simulink model "AircraftModel_LonMot_SAS"  (R2023b)
settings: Solver=VariableStepAuto  StartTime=0.0  StopTime=150  FixedStep=CNT_StepSize  RelTol=1e-3
undefined symbols (not defined in the file or in its folder): Actuators, CNT_g, CNT_m, ControlLaws, Propulsion, TestSequence, TrimPoint
libraries: simulink x6, vrlib x2
settings Model: Creator=NicolasS  LastModifiedBy=rouve
settings SolverCC: AlgebraicLoopSolver=TrustRegion
settings DataIOCC: ExternalInput=getinputstruct(TrimState_1_Op)  InitialState=getstatestruct(TrimState_1_Op)
settings DebuggingCC: UnconnectedInputMsg=warning  UnconnectedOutputMsg=warning  UnconnectedLineMsg=warning
settings ModelReferenceCC: EnableRefExpFcnMdlSchedulingChecks=on
settings RTWCC: DLArmComputeVersion=19.05

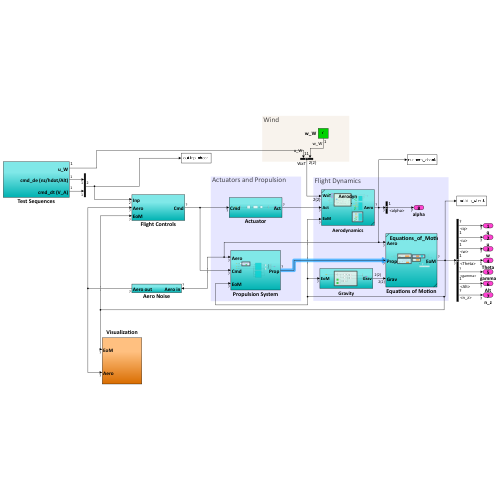
[thumbnail: Simulink's stored preview of the top-level diagram]
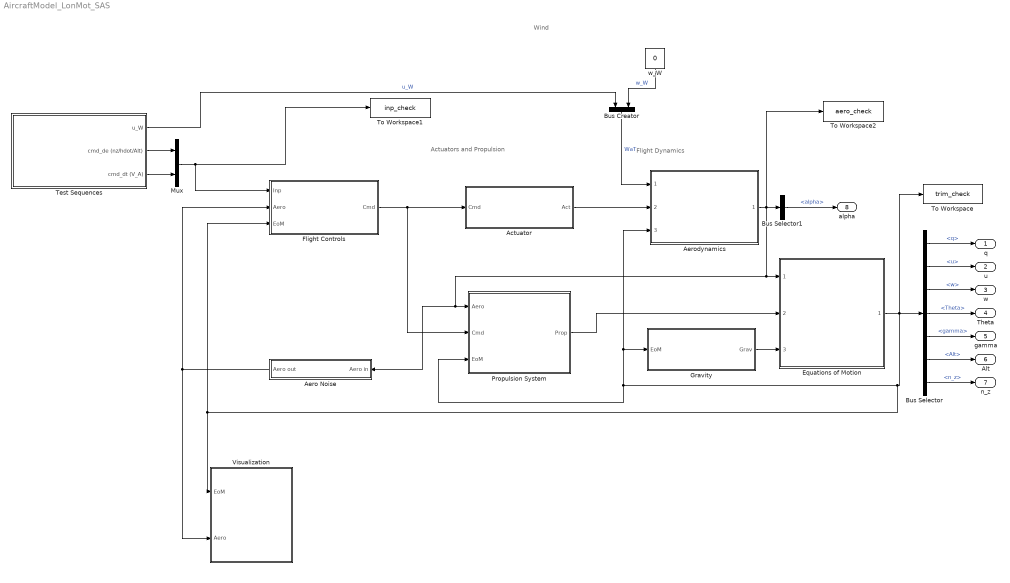
== system AircraftModel_LonMot_SAS ==
  note: Wind
  note: Actuators and Propulsion
  note: Flight Dynamics
  Actuator : Subsystem
  Aero Noise : Subsystem
  Aerodynamics : Subsystem  ReferencedSubsystem=Aerodyn
  Bus Creator : BusCreator  Inputs=2  OutDataTypeStr=Bus: WaT
  Bus Selector : BusSelector  OutputSignals=q,vv_f.u,vv_f.w,Theta,gamma,Alt,nn_f.n_z
  Bus Selector1 : BusSelector  OutputSignals=AirData.alpha
  Equations of Motion : Subsystem  ReferencedSubsystem=Equations_of_Motion
  Flight Controls : Subsystem
  Gravity : Subsystem
  Mux : Mux  Inputs=2
  Propulsion System : Subsystem
  Test Sequences : Subsystem  InitFcn=|  StopFcn=clear TestSequence
      | if not(exist('TestSequence','var'))
      |        TestSequence = 0;
      | end
  To Workspace : ToWorkspace  VariableName=trim_check  SaveFormat=Timeseries  SampleTime=-1
      settings: Decimation=2
  To Workspace1 : ToWorkspace  VariableName=inp_check  SaveFormat=Timeseries  SampleTime=-1
  To Workspace2 : ToWorkspace  VariableName=aero_check  SaveFormat=Timeseries  SampleTime=-1
  Visualization : Subsystem
  w_W : Constant  Value=0  SampleTime=-1
  q : Outport
  u : Outport  Port=2
  w : Outport  Port=3
  Theta : Outport  Port=4
  gamma : Outport  Port=5
  Alt : Outport  Port=6
  n_z : Outport  Port=7
  alpha : Outport  Port=8
  wires:
  Test Sequences/1(u_W) -> Bus Creator/1  "u_W"
  Bus Creator/1 -> Aerodynamics/1  "WaT"
  Actuator/1(Act) -> Aerodynamics/2
  Aerodynamics/1 -> To Workspace2/1, Bus Selector1/1, Propulsion System/1(Aero), Aero Noise/1(Aero in), Equations of Motion/1
  w_W/1 -> Bus Creator/2  "w_W"
  Propulsion System/1(Prop) -> Equations of Motion/2
  Bus Selector/6 -> Alt/1  "<Alt>"
  Bus Selector/1 -> q/1  "<q>"
  Bus Selector/2 -> u/1  "<u>"
  Bus Selector/3 -> w/1  "<w>"
  Bus Selector/4 -> Theta/1  "<Theta>"
  Bus Selector/7 -> n_z/1  "<n_z>"
  Bus Selector1/1 -> alpha/1  "<alpha>"
  Gravity/1(Grav) -> Equations of Motion/3
  Bus Selector/5 -> gamma/1  "<gamma>"
  Aero Noise/1(Aero out) -> Visualization/2(Aero), Flight Controls/2(Aero)
  Test Sequences/2(cmd_de (nz/hdot/Alt)) -> Mux/1
  Test Sequences/3(cmd_dt (V_A)) -> Mux/2
  Mux/1 -> Flight Controls/1(Inp), To Workspace1/1
  Flight Controls/1(Cmd) -> Propulsion System/2(Cmd), Actuator/1(Cmd)
  Equations of Motion/1 -> To Workspace/1, Visualization/1(EoM), Flight Controls/3(EoM), Propulsion System/3(EoM), Aerodynamics/3, Gravity/1(EoM), Bus Selector/1

== system AircraftModel_LonMot_SAS/Actuator ==
  Cmd : Inport  OutDataTypeStr=Bus: Cmd
  Bus Creator : BusCreator  Inputs=1  OutDataTypeStr=Bus: Act
  Bus Selector : BusSelector  OutputSignals=cmd_de
  Saturation : Saturate  UpperLimit=Actuators.Limits.u_max_He(2)  LowerLimit=Actuators.Limits.u_max_He(1)
  State-Space : StateSpace  A=Actuators.Act_e.A  B=Actuators.Act_e.B  C=Actuators.Act_e.C  D=Actuators.Act_e.D  InitialCondition=TrimPoint.States.debar  ParameterTunability=Unconstrained  ContinuousStateAttributes='de'
  Transport Delay : TransportDelay  DelayTime=0.04  InitialOutput=TrimPoint.States.debar  TransDelayFeedthrough=on
  Act : Outport  OutDataTypeStr=Bus: Act
  wires:
  Bus Creator/1 -> Act/1  "Act"
  Cmd/1 -> Bus Selector/1
  State-Space/1 -> Saturation/1  "de"
  Bus Selector/1 -> Transport Delay/1  "<cmd_de>"
  Saturation/1 -> Bus Creator/1  "de"
  Transport Delay/1 -> State-Space/1

== system AircraftModel_LonMot_SAS/Aero Noise ==
  Aero in : Inport  OutDataTypeStr=Bus: Aero
  Band-Limited White Noise8 : simulink/Sources/Band-Limited White Noise  Cov=1E-7  Ts=0.01  seed=3324
  Band-Limited White Noise9 : simulink/Sources/Band-Limited White Noise  Cov=1E-3  Ts=0.05  seed=8153
  Bus Creator2 : BusCreator  Inputs=4  OutDataTypeStr=Bus: Aero
  Bus Creator3 : BusCreator  Inputs=5  OutDataTypeStr=Bus: AirData
  Bus Selector : BusSelector  OutputSignals=AirData.u_Af,AirData.w_Af,AirData.V_A,AirData.p_dyn,AirData.alpha,X_Af,Z_Af,M_Af
  Sum1 : Sum  Inputs=++|
  Sum3 : Sum  Inputs=++|
  Aero out : Outport  OutDataTypeStr=Bus: Aero
  wires:
  Aero in/1 -> Bus Selector/1
  Bus Creator3/1 -> Bus Creator2/1  "AirData"
  Bus Selector/6 -> Bus Creator2/2  "<X_Af>"
  Bus Selector/7 -> Bus Creator2/3  "<Z_Af>"
  Bus Selector/8 -> Bus Creator2/4  "<M_Af>"
  Bus Creator2/1 -> Aero out/1  "Aero"
  Bus Selector/1 -> Bus Creator3/1  "<u_Af>"
  Bus Selector/2 -> Bus Creator3/2  "<w_Af>"
  Bus Selector/3 -> Sum3/2  "<V_A>"
  Bus Selector/5 -> Sum1/2  "<alpha>"
  Band-Limited White Noise8/1 -> Sum1/1
  Sum1/1 -> Bus Creator3/5  "alpha"
  Bus Selector/4 -> Bus Creator3/4  "<p_dyn>"
  Band-Limited White Noise9/1 -> Sum3/1
  Sum3/1 -> Bus Creator3/3  "V_A"

== system AircraftModel_LonMot_SAS/Flight Controls ==
  Inp : Inport
  Aero : Inport  Port=2  OutDataTypeStr=Bus: Aero
  EoM : Inport  Port=3  OutDataTypeStr=Bus: EoM
  Bus Creator2 : BusCreator  Inputs=2  OutDataTypeStr=Bus: Cmd
  Longitudinal Control Laws : Subsystem
  Cmd : Outport
  wires:
  EoM/1 -> Longitudinal Control Laws/2(EoM)
  Bus Creator2/1 -> Cmd/1  "Cmd"
  Longitudinal Control Laws/2(cmd_dt) -> Bus Creator2/2  "cmd_dt"
  Longitudinal Control Laws/1(cmd_de) -> Bus Creator2/1  "cmd_de"
  Inp/1 -> Longitudinal Control Laws/3(Inp)
  Aero/1 -> Longitudinal Control Laws/1(Aero)

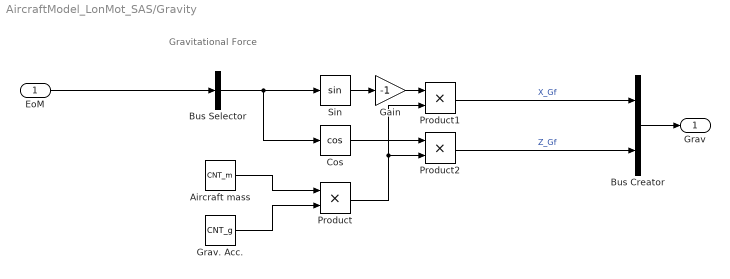
== system AircraftModel_LonMot_SAS/Gravity ==
  note: Gravitational Force
  EoM : Inport  OutDataTypeStr=Bus: EoM
  Aircraft mass : Constant  Value=CNT_m  SampleTime=-1
  Bus Creator : BusCreator  Inputs=2  OutDataTypeStr=Bus: Grav
  Bus Selector : BusSelector  OutputSignals=Theta  OutputAsBus=on
  Cos : Trigonometry  Operator=cos
  Gain : Gain  Gain=-1
  Grav. Acc. : Constant  Value=CNT_g  SampleTime=-1
  Product : Product
  Product1 : Product
  Product2 : Product
  Sin : Trigonometry
  Grav : Outport  OutDataTypeStr=Bus: Grav
  wires:
  EoM/1 -> Bus Selector/1
  Product1/1 -> Bus Creator/1  "X_Gf"
  Product2/1 -> Bus Creator/2  "Z_Gf"
  Bus Creator/1 -> Grav/1
  Aircraft mass/1 -> Product/1
  Grav. Acc./1 -> Product/2
  Bus Selector/1 -> Cos/1, Sin/1
  Sin/1 -> Gain/1
  Gain/1 -> Product1/1
  Cos/1 -> Product2/1
  Product/1 -> Product2/2, Product1/2

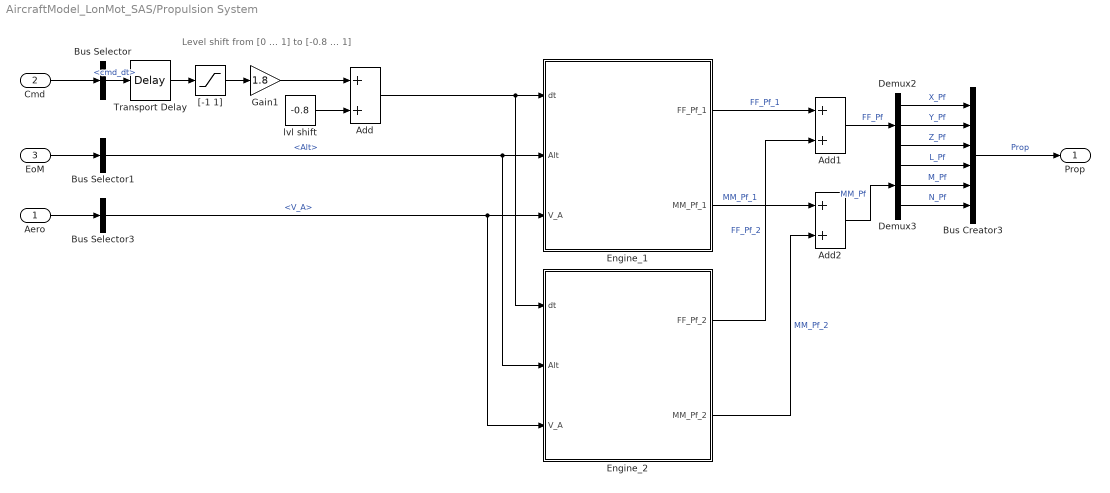
== system AircraftModel_LonMot_SAS/Propulsion System ==
  note: Level shift from [0 ... 1] to [-0.8 ... 1]
  Aero : Inport  OutDataTypeStr=Bus: Aero
  Cmd : Inport  Port=2  OutDataTypeStr=Bus: Cmd
  EoM : Inport  Port=3  OutDataTypeStr=Bus: EoM
  Add : Sum
  Add1 : Sum
  Add2 : Sum
  Bus Creator3 : BusCreator  Inputs=6  OutDataTypeStr=Bus: Prop
  Bus Selector : BusSelector  OutputSignals=cmd_dt
  Bus Selector1 : BusSelector  OutputSignals=Alt
  Bus Selector3 : BusSelector  OutputSignals=AirData.V_A
  Demux2 : Demux  Outputs=3
  Demux3 : Demux  Outputs=3
  Engine_1 : Subsystem
  Engine_2 : Subsystem
  Gain1 : Gain  Gain=1.8
  Transport Delay : TransportDelay  DelayTime=Propulsion.Act_t.InputDelay  InitialOutput=TrimPoint.States.dtbar  TransDelayFeedthrough=on
  "[-1 1]" : Saturate  UpperLimit=1  LowerLimit=0
  lvl shift : Constant  Value=-0.8  SampleTime=-1
  Prop : Outport  OutDataTypeStr=Bus: Prop
  wires:
  Demux2/2 -> Bus Creator3/2  "Y_Pf"
  Engine_1/1(FF_Pf_1) -> Add1/1  "FF_Pf_1"
  Demux3/1 -> Bus Creator3/4  "L_Pf"
  EoM/1 -> Bus Selector1/1
  lvl shift/1 -> Add/2
  Engine_2/1(FF_Pf_2) -> Add1/2  "FF_Pf_2"
  Add2/1 -> Demux3/1  "MM_Pf"
  Bus Selector3/1 -> Engine_2/3(V_A), Engine_1/3(V_A)  "<V_A>"
  Aero/1 -> Bus Selector3/1
  Demux2/1 -> Bus Creator3/1  "X_Pf"
  Gain1/1 -> Add/1
  Engine_1/2(MM_Pf_1) -> Add2/1  "MM_Pf_1"
  Add/1 -> Engine_2/1(dt), Engine_1/1(dt)
  Bus Creator3/1 -> Prop/1  "Prop"
  Demux3/2 -> Bus Creator3/5  "M_Pf"
  "[-1 1]"/1 -> Gain1/1
  Demux2/3 -> Bus Creator3/3  "Z_Pf"
  Add1/1 -> Demux2/1  "FF_Pf"
  Bus Selector1/1 -> Engine_2/2(Alt), Engine_1/2(Alt)  "<Alt>"
  Demux3/3 -> Bus Creator3/6  "N_Pf"
  Cmd/1 -> Bus Selector/1
  Bus Selector/1 -> Transport Delay/1  "<cmd_dt>"
  Engine_2/2(MM_Pf_2) -> Add2/2  "MM_Pf_2"
  Transport Delay/1 -> "[-1 1]"/1

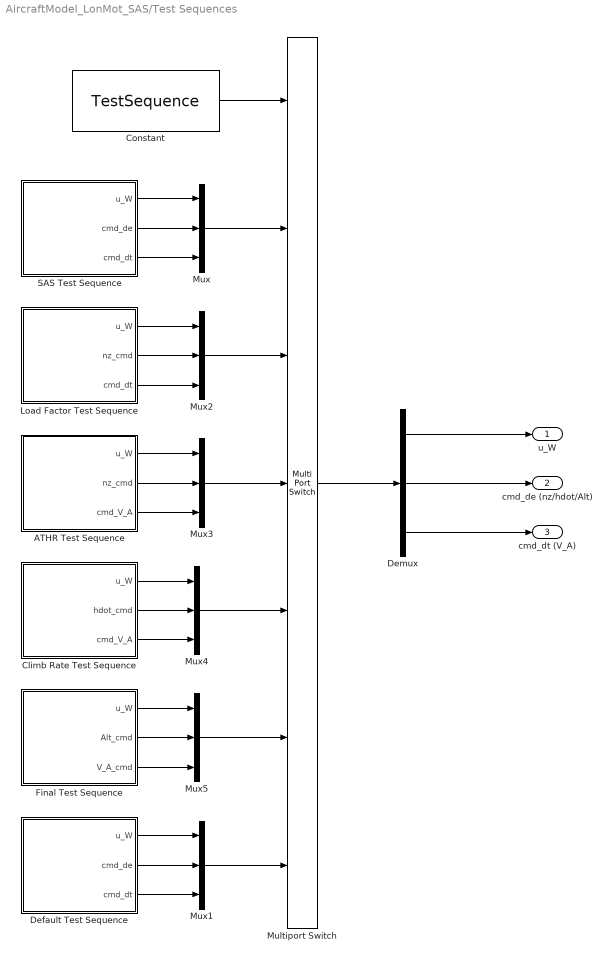
== system AircraftModel_LonMot_SAS/Test Sequences ==
  ATHR Test Sequence : Subsystem
  Climb Rate Test Sequence : Subsystem
  Constant : Constant  Value=TestSequence
  Default Test Sequence : Subsystem
  Demux : Demux  Outputs=3
  Final Test Sequence : Subsystem
  Load Factor Test Sequence : Subsystem
  Multiport Switch : MultiPortSwitch  Inputs=6  SaturateOnIntegerOverflow=off  InputSameDT=off
  Mux{,1..5} (6 alike) : Mux  Inputs=3
  SAS Test Sequence : Subsystem
  u_W : Outport
  cmd_de (nz/hdot/Alt) : Outport  Port=2
  cmd_dt (V_A) : Outport  Port=3
  wires:
  Demux/1 -> u_W/1
  Demux/2 -> cmd_de (nz/hdot/Alt)/1
  Demux/3 -> cmd_dt (V_A)/1
  Constant/1 -> Multiport Switch/1
  SAS Test Sequence/1(u_W) -> Mux/1
  SAS Test Sequence/2(cmd_de) -> Mux/2
  SAS Test Sequence/3(cmd_dt) -> Mux/3
  Mux/1 -> Multiport Switch/2
  Multiport Switch/1 -> Demux/1
  Default Test Sequence/1(u_W) -> Mux1/1
  Default Test Sequence/2(cmd_de) -> Mux1/2
  Default Test Sequence/3(cmd_dt) -> Mux1/3
  Mux1/1 -> Multiport Switch/7
  Load Factor Test Sequence/1(u_W) -> Mux2/1
  Load Factor Test Sequence/2(nz_cmd) -> Mux2/2
  Load Factor Test Sequence/3(cmd_dt) -> Mux2/3
  Mux2/1 -> Multiport Switch/3
  ATHR Test Sequence/1(u_W) -> Mux3/1
  ATHR Test Sequence/2(nz_cmd) -> Mux3/2
  ATHR Test Sequence/3(cmd_V_A) -> Mux3/3
  Mux3/1 -> Multiport Switch/4
  Climb Rate Test Sequence/1(u_W) -> Mux4/1
  Climb Rate Test Sequence/2(hdot_cmd) -> Mux4/2
  Climb Rate Test Sequence/3(cmd_V_A) -> Mux4/3
  Mux4/1 -> Multiport Switch/5
  Final Test Sequence/1(u_W) -> Mux5/1
  Final Test Sequence/2(Alt_cmd) -> Mux5/2
  Final Test Sequence/3(V_A_cmd) -> Mux5/3
  Mux5/1 -> Multiport Switch/6

== system AircraftModel_LonMot_SAS/Visualization ==
  EoM : Inport  OutDataTypeStr=Bus: EoM
  Aero : Inport  Port=2  OutDataTypeStr=Bus: Aero
  Bus Selector2 : BusSelector  OutputSignals=q,vv_f.u,vv_f.w,Theta,Alt,nn_f.n_z
  Bus Selector3 : BusSelector  OutputSignals=AirData.alpha
  Gain11 : Gain  Gain=180/pi
  Gain8 : Gain  Gain=180/pi
  Gain9 : Gain  Gain=180/pi
  Scope2 : Scope  NumInputPorts=7
  wires:
  Gain8/1 -> Scope2/2  "q"
  Gain11/1 -> Scope2/1  "alpha"
  Gain9/1 -> Scope2/5  "Theta"
  Aero/1 -> Bus Selector3/1
  Bus Selector2/2 -> Scope2/3  "<u>"
  Bus Selector2/1 -> Gain8/1  "<q>"
  EoM/1 -> Bus Selector2/1
  Bus Selector2/6 -> Scope2/7  "<n_z>"
  Bus Selector2/5 -> Scope2/6  "<Alt>"
  Bus Selector3/1 -> Gain11/1  "<alpha>"
  Bus Selector2/3 -> Scope2/4  "<w>"
  Bus Selector2/4 -> Gain9/1  "<Theta>"

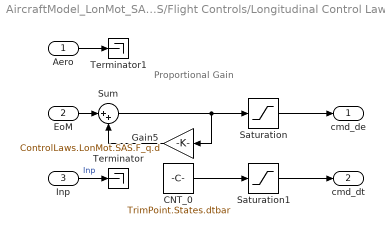
== system AircraftModel_LonMot_SAS/Flight Controls/Longitudinal Control Laws ==
  note: Proportional
      | Gain
  Aero : Inport  OutDataTypeStr=Bus: Aero
  EoM : Inport  Port=2  OutDataTypeStr=Bus: EoM
  Inp : Inport  Port=3
  CNT_0 : Constant  Value=TrimPoint.States.dtbar
  Gain5 : Gain  Gain=ControlLaws.LonMot.SAS.F_q.d
  Saturation : Saturate  UpperLimit=Actuators.Limits.u_max_He(2)  LowerLimit=Actuators.Limits.u_max_He(1)
  Saturation1 : Saturate  UpperLimit=1  LowerLimit=0
  Sum : Sum  Inputs=|++
  Terminator : Terminator
  Terminator1 : Terminator
  cmd_de : Outport
  cmd_dt : Outport  Port=2
  wires:
  Inp/1 -> Terminator/1  "Inp"
  Aero/1 -> Terminator1/1
  Saturation/1 -> cmd_de/1
  CNT_0/1 -> Saturation1/1
  Saturation1/1 -> cmd_dt/1
  EoM/1 -> Sum/1
  Gain5/1 -> Sum/2
  Sum/1 -> Gain5/1, Saturation/1

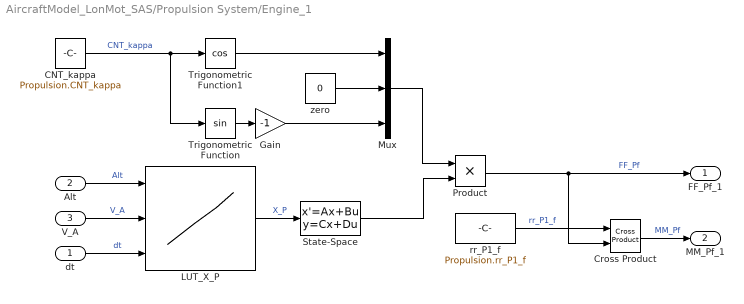
== system AircraftModel_LonMot_SAS/Propulsion System/Engine_1 ==
  dt : Inport
  Alt : Inport  Port=2
  V_A : Inport  Port=3
  CNT_kappa : Constant  Value=Propulsion.CNT_kappa  SampleTime=-1
  Cross Product : vrlib/Utilities/Cross Product
  Gain : Gain  Gain=-1
  LUT_X_P : Lookup_n-D  NumberOfTableDimensions=3  BreakpointsForDimension1=Propulsion.LUT.LUT_Alt  BreakpointsForDimension2=Propulsion.LUT.LUT_V_A  BreakpointsForDimension3=Propulsion.LUT.LUT_dt  Table=Propulsion.LUT.LUT_X_P  ExtrapMethod=Clip
      settings: InputPortMap=u0,u1,u2
  Mux : Mux  Inputs=3
  Product : Product  RndMeth=Zero
  State-Space : StateSpace  A=Propulsion.Act_t.A  B=Propulsion.Act_t.B  C=Propulsion.Act_t.C  D=Propulsion.Act_t.D  InitialCondition=TrimPoint.States.X_P  ParameterTunability=Unconstrained  ContinuousStateAttributes='X_P1'
  Trigonometric Function : Trigonometry
  Trigonometric Function1 : Trigonometry  Operator=cos
  "rr_P1_f " : Constant  Value=Propulsion.rr_P1_f  SampleTime=-1
  zero : Constant  Value=0  SampleTime=-1
  FF_Pf_1 : Outport
  MM_Pf_1 : Outport  Port=2
  wires:
  Alt/1 -> LUT_X_P/1  "Alt"
  V_A/1 -> LUT_X_P/2  "V_A"
  dt/1 -> LUT_X_P/3  "dt"
  zero/1 -> Mux/2
  Mux/1 -> Product/1
  CNT_kappa/1 -> Trigonometric Function1/1, Trigonometric Function/1  "CNT_kappa"
  Trigonometric Function1/1 -> Mux/1
  Product/1 -> FF_Pf_1/1, Cross Product/2  "FF_Pf"
  Cross Product/1 -> MM_Pf_1/1  "MM_Pf"
  Trigonometric Function/1 -> Gain/1
  Gain/1 -> Mux/3
  LUT_X_P/1 -> State-Space/1  "X_P"
  "rr_P1_f "/1 -> Cross Product/1  "rr_P1_f"
  State-Space/1 -> Product/2

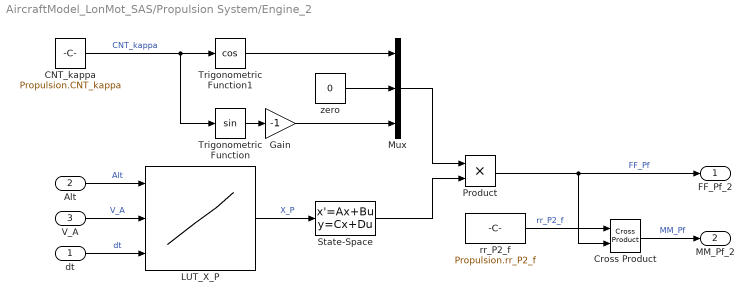
== system AircraftModel_LonMot_SAS/Propulsion System/Engine_2 ==
  dt : Inport
  Alt : Inport  Port=2
  V_A : Inport  Port=3
  CNT_kappa : Constant  Value=Propulsion.CNT_kappa  SampleTime=-1
  Cross Product : vrlib/Utilities/Cross Product
  Gain : Gain  Gain=-1
  LUT_X_P : Lookup_n-D  NumberOfTableDimensions=3  BreakpointsForDimension1=Propulsion.LUT.LUT_Alt  BreakpointsForDimension2=Propulsion.LUT.LUT_V_A  BreakpointsForDimension3=Propulsion.LUT.LUT_dt  Table=Propulsion.LUT.LUT_X_P
      settings: InputPortMap=u0,u1,u2
  Mux : Mux  Inputs=3
  Product : Product  RndMeth=Zero
  State-Space : StateSpace  A=Propulsion.Act_t.A  B=Propulsion.Act_t.B  C=Propulsion.Act_t.C  D=Propulsion.Act_t.D  InitialCondition=TrimPoint.States.X_P  ParameterTunability=Unconstrained  ContinuousStateAttributes='X_P2'
  Trigonometric Function : Trigonometry
  Trigonometric Function1 : Trigonometry  Operator=cos
  "rr_P2_f " : Constant  Value=Propulsion.rr_P2_f  SampleTime=-1
  zero : Constant  Value=0  SampleTime=-1
  FF_Pf_2 : Outport
  MM_Pf_2 : Outport  Port=2
  wires:
  zero/1 -> Mux/2
  Gain/1 -> Mux/3
  Mux/1 -> Product/1
  Cross Product/1 -> MM_Pf_2/1  "MM_Pf"
  Trigonometric Function1/1 -> Mux/1
  Product/1 -> FF_Pf_2/1, Cross Product/2  "FF_Pf"
  Trigonometric Function/1 -> Gain/1
  Alt/1 -> LUT_X_P/1  "Alt"
  dt/1 -> LUT_X_P/3  "dt"
  LUT_X_P/1 -> State-Space/1  "X_P"
  V_A/1 -> LUT_X_P/2  "V_A"
  "rr_P2_f "/1 -> Cross Product/1  "rr_P2_f"
  CNT_kappa/1 -> Trigonometric Function1/1, Trigonometric Function/1  "CNT_kappa"
  State-Space/1 -> Product/2

== system AircraftModel_LonMot_SAS/Test Sequences/ATHR Test Sequence ==
  Add : Sum
  Constant1 : Constant  Value=0
  Constant2 : Constant  Value=sqrt(TrimPoint.States.ubar^2+TrimPoint.States.wbar^2)
  Doublet Generator : Subsystem  mask(DoubletGenerator){timeon=5, pulsewidth=30, amplitude=10}
      mask prompts: timeon "Time Start"; pulsewidth "Pulse Duration"
      mask help:
      | Doublet Generator.
      | Ouputs doublet of specificed amplitude and duration.
      |
      | If start/duration/amplitude parameters are vectors, then output is multichannel.
      mask Display: plot([.1 .3 .3001 .4 .4001 .5  .5001 .7],[0 0 1 1 -1 -1 0 0])
  Gust Generator : Subsystem  mask{gust_start=100, gust_duration=15, gust_amplitude=20}
      mask prompts: gust_start "start time of the gust in sec"; gust_duration "gust duration in sec"; gust_amplitude "maximum gust speed in m/s"
      mask DialogControl ParameterGroupVar Prompt: gust characteristics
  u_W : Outport  PortDimensions=1
  nz_cmd : Outport  Port=2
  cmd_V_A : Outport  Port=3
  wires:
  Constant1/1 -> nz_cmd/1  "nz_cmd"
  Doublet Generator/1(Doublet) -> Add/1
  Gust Generator/1(wind speed) -> u_W/1  "u_W"
  Add/1 -> cmd_V_A/1  "cmd_V_A"
  Constant2/1 -> Add/2  "nz_cmd"

== system AircraftModel_LonMot_SAS/Test Sequences/Climb Rate Test Sequence ==
  Constant1 : Constant  Value=0
  Constant2 : Constant  Value=sqrt(TrimPoint.States.ubar^2+TrimPoint.States.wbar^2)
  Doublet Generator : Subsystem  mask(DoubletGenerator){timeon=5, pulsewidth=20, amplitude=5}
      mask prompts: timeon "Time Start"; pulsewidth "Pulse Duration"
      mask help:
      | Doublet Generator.
      | Ouputs doublet of specificed amplitude and duration.
      |
      | If start/duration/amplitude parameters are vectors, then output is multichannel.
      mask Display: plot([.1 .3 .3001 .4 .4001 .5  .5001 .7],[0 0 1 1 -1 -1 0 0])
  u_W : Outport  PortDimensions=1
  hdot_cmd : Outport  Port=2
  cmd_V_A : Outport  Port=3
  wires:
  Doublet Generator/1(Doublet) -> hdot_cmd/1  "hdot_cmd"
  Constant1/1 -> u_W/1  "u_W"
  Constant2/1 -> cmd_V_A/1  "cmd_V_A"

== system AircraftModel_LonMot_SAS/Test Sequences/Default Test Sequence ==
  Constant : Constant  Value=TrimPoint.States.debar
  Constant1 : Constant  Value=0
  Constant2 : Constant  Value=TrimPoint.States.dtbar
  u_W : Outport  PortDimensions=1
  cmd_de : Outport  Port=2
  cmd_dt : Outport  Port=3
  wires:
  Constant/1 -> cmd_de/1  "cmd_de"
  Constant2/1 -> cmd_dt/1  "cmd_dt"
  Constant1/1 -> u_W/1  "u_W"

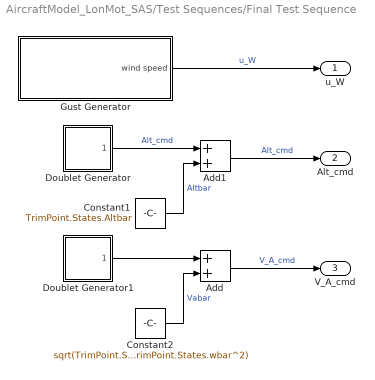
== system AircraftModel_LonMot_SAS/Test Sequences/Final Test Sequence ==
  Add : Sum
  Add1 : Sum
  Constant1 : Constant  Value=TrimPoint.States.Altbar
  Constant2 : Constant  Value=sqrt(TrimPoint.States.ubar^2+TrimPoint.States.wbar^2)
  Doublet Generator : Subsystem  mask(DoubletGenerator){timeon=5, pulsewidth=40, amplitude=100}
      mask prompts: timeon "Time Start"; pulsewidth "Pulse Duration"
      mask help:
      | Doublet Generator.
      | Ouputs doublet of specificed amplitude and duration.
      |
      | If start/duration/amplitude parameters are vectors, then output is multichannel.
      mask Display: plot([.1 .3 .3001 .4 .4001 .5  .5001 .7],[0 0 1 1 -1 -1 0 0])
  Doublet Generator1 : Subsystem  mask(DoubletGenerator){timeon=5, pulsewidth=60, amplitude=10}
      mask prompts: timeon "Time Start"; pulsewidth "Pulse Duration"
      mask help:
      | Doublet Generator.
      | Ouputs doublet of specificed amplitude and duration.
      |
      | If start/duration/amplitude parameters are vectors, then output is multichannel.
      mask Display: plot([.1 .3 .3001 .4 .4001 .5  .5001 .7],[0 0 1 1 -1 -1 0 0])
  Gust Generator : Subsystem  mask{gust_start=30, gust_duration=15, gust_amplitude=20}
      mask prompts: gust_start "start time of the gust in sec"; gust_duration "gust duration in sec"; gust_amplitude "maximum gust speed in m/s"
      mask DialogControl ParameterGroupVar Prompt: gust characteristics
  u_W : Outport  PortDimensions=1
  Alt_cmd : Outport  Port=2
  V_A_cmd : Outport  Port=3
  wires:
  Doublet Generator/1(Doublet) -> Add1/1  "Alt_cmd"
  Gust Generator/1(wind speed) -> u_W/1  "u_W"
  Add/1 -> V_A_cmd/1  "V_A_cmd"
  Doublet Generator1/1(Doublet) -> Add/1
  Constant2/1 -> Add/2  "Vabar"
  Constant1/1 -> Add1/2  "Altbar"
  Add1/1 -> Alt_cmd/1  "Alt_cmd"

== system AircraftModel_LonMot_SAS/Test Sequences/Load Factor Test Sequence ==
  Constant2 : Constant  Value=TrimPoint.States.dtbar
  Doublet Generator : Subsystem  mask(DoubletGenerator){timeon=5, pulsewidth=6, amplitude=0.2}
      mask prompts: timeon "Time Start"; pulsewidth "Pulse Duration"
      mask help:
      | Doublet Generator.
      | Ouputs doublet of specificed amplitude and duration.
      |
      | If start/duration/amplitude parameters are vectors, then output is multichannel.
      mask Display: plot([.1 .3 .3001 .4 .4001 .5  .5001 .7],[0 0 1 1 -1 -1 0 0])
  Gust Generator : Subsystem  mask{gust_start=20, gust_duration=15, gust_amplitude=20}
      mask prompts: gust_start "start time of the gust in sec"; gust_duration "gust duration in sec"; gust_amplitude "maximum gust speed in m/s"
      mask DialogControl ParameterGroupVar Prompt: gust characteristics
  u_W : Outport  PortDimensions=1
  nz_cmd : Outport  Port=2
  cmd_dt : Outport  Port=3
  wires:
  Doublet Generator/1(Doublet) -> nz_cmd/1  "nz_cmd"
  Constant2/1 -> cmd_dt/1  "cmd_dt"
  Gust Generator/1(wind speed) -> u_W/1  "u_W"

== system AircraftModel_LonMot_SAS/Test Sequences/SAS Test Sequence ==
  Constant2 : Constant  Value=TrimPoint.States.dtbar
  Gust Generator : Subsystem  mask{gust_start=15, gust_duration=15, gust_amplitude=20}
      mask prompts: gust_start "start time of the gust in sec"; gust_duration "gust duration in sec"; gust_amplitude "maximum gust speed in m/s"
      mask DialogControl ParameterGroupVar Prompt: gust characteristics
  Step : Step  Time=5  Before=TrimPoint.States.debar  After=TrimPoint.States.debar + deg2rad(-1)  SampleTime=0
  u_W : Outport  PortDimensions=1
  cmd_de : Outport  Port=2
  cmd_dt : Outport  Port=3
  wires:
  Step/1 -> cmd_de/1  "cmd_de"
  Constant2/1 -> cmd_dt/1  "cmd_dt"
  Gust Generator/1(wind speed) -> u_W/1  "u_W"

== system AircraftModel_LonMot_SAS/Test Sequences/ATHR Test Sequence/Doublet Generator ==
  Add : Sum  Inputs=+++
  DownStep : Step  Time=timeon+pulsewidth  After=-1  SampleTime=0
  Gain : Gain  Gain=amplitude
  UnStep : Step  Time=timeon+2*pulsewidth  After=-1  SampleTime=0
  UpStep : Step  Time=timeon  SampleTime=0
  Doublet : Outport
  wires:
  UpStep/1 -> Add/1
  DownStep/1 -> Add/2
  UnStep/1 -> Add/3
  Add/1 -> Gain/1
  Gain/1 -> Doublet/1

== system AircraftModel_LonMot_SAS/Test Sequences/ATHR Test Sequence/Gust Generator ==
  1-cos gust : Subsystem  TreatAsAtomicUnit=on
  Clock : Clock
  Compare To Constant : simulink/Logic and Bit Operations/Compare To Constant  relop=>=  const=gust_start  OutDataTypeStr=boolean
  Constant : Constant  Value=0
  Sum : Sum  Inputs=+-|
  Switch : Switch  Criteria=u2 > Threshold  Threshold=gust_start+gust_duration  SaturateOnIntegerOverflow=off  InputSameDT=off
  time freeze : Subsystem  TreatAsAtomicUnit=on
  wind speed : Outport
  wires:
  time freeze/1(out) -> Sum/2
  Constant/1 -> Switch/1
  Clock/1 -> time freeze/1(in), Compare To Constant/1, Sum/1, Switch/2
  Compare To Constant/1 -> 1-cos gust/Enable, time freeze/Trigger
  Sum/1 -> 1-cos gust/1(in)
  1-cos gust/1(wind) -> Switch/3
  Switch/1 -> wind speed/1

== system AircraftModel_LonMot_SAS/Test Sequences/Climb Rate Test Sequence/Doublet Generator ==
  Add : Sum  Inputs=+++
  DownStep : Step  Time=timeon+pulsewidth  After=-2  SampleTime=0
  Gain : Gain  Gain=amplitude
  UnStep : Step  Time=timeon+2*pulsewidth  SampleTime=0
  UpStep : Step  Time=timeon  SampleTime=0
  Doublet : Outport
  wires:
  UpStep/1 -> Add/1
  DownStep/1 -> Add/2
  UnStep/1 -> Add/3
  Add/1 -> Gain/1
  Gain/1 -> Doublet/1

== system AircraftModel_LonMot_SAS/Test Sequences/Final Test Sequence/Doublet Generator ==
  Add : Sum  Inputs=+++
  DownStep : Step  Time=timeon+pulsewidth  After=-2  SampleTime=0
  Gain : Gain  Gain=amplitude
  UnStep : Step  Time=timeon+2*pulsewidth  SampleTime=0
  UpStep : Step  Time=timeon  SampleTime=0
  Doublet : Outport
  wires:
  UpStep/1 -> Add/1
  DownStep/1 -> Add/2
  UnStep/1 -> Add/3
  Add/1 -> Gain/1
  Gain/1 -> Doublet/1

== system AircraftModel_LonMot_SAS/Test Sequences/Final Test Sequence/Doublet Generator1 ==
  Add : Sum  Inputs=+++
  DownStep : Step  Time=timeon+pulsewidth  SampleTime=0
  Gain : Gain  Gain=amplitude
  UnStep : Step  Time=timeon+2*pulsewidth  After=-1  SampleTime=0
  UpStep : Step  Time=timeon  SampleTime=0
  Doublet : Outport
  wires:
  UpStep/1 -> Add/1
  DownStep/1 -> Add/2
  UnStep/1 -> Add/3
  Add/1 -> Gain/1
  Gain/1 -> Doublet/1

== system AircraftModel_LonMot_SAS/Test Sequences/Final Test Sequence/Gust Generator ==
  1-cos gust : Subsystem  TreatAsAtomicUnit=on
  Clock : Clock
  Compare To Constant : simulink/Logic and Bit Operations/Compare To Constant  relop=>=  const=gust_start  OutDataTypeStr=boolean
  Constant : Constant  Value=0
  Sum : Sum  Inputs=+-|
  Switch : Switch  Criteria=u2 > Threshold  Threshold=gust_start+gust_duration  SaturateOnIntegerOverflow=off  InputSameDT=off
  time freeze : Subsystem  TreatAsAtomicUnit=on
  wind speed : Outport
  wires:
  time freeze/1(out) -> Sum/2
  Constant/1 -> Switch/1
  Clock/1 -> time freeze/1(in), Compare To Constant/1, Sum/1, Switch/2
  Compare To Constant/1 -> 1-cos gust/Enable, time freeze/Trigger
  Sum/1 -> 1-cos gust/1(in)
  1-cos gust/1(wind) -> Switch/3
  Switch/1 -> wind speed/1

== system AircraftModel_LonMot_SAS/Test Sequences/Load Factor Test Sequence/Doublet Generator ==
  Add : Sum  Inputs=+++
  DownStep : Step  Time=timeon+pulsewidth  After=-2  SampleTime=0
  Gain : Gain  Gain=amplitude
  UnStep : Step  Time=timeon+2*pulsewidth  SampleTime=0
  UpStep : Step  Time=timeon  SampleTime=0
  Doublet : Outport
  wires:
  UpStep/1 -> Add/1
  DownStep/1 -> Add/2
  UnStep/1 -> Add/3
  Add/1 -> Gain/1
  Gain/1 -> Doublet/1

== system AircraftModel_LonMot_SAS/Test Sequences/Load Factor Test Sequence/Gust Generator ==
  1-cos gust : Subsystem  TreatAsAtomicUnit=on
  Clock : Clock
  Compare To Constant : simulink/Logic and Bit Operations/Compare To Constant  relop=>=  const=gust_start  OutDataTypeStr=boolean
  Constant : Constant  Value=0
  Sum : Sum  Inputs=+-|
  Switch : Switch  Criteria=u2 > Threshold  Threshold=gust_start+gust_duration  SaturateOnIntegerOverflow=off  InputSameDT=off
  time freeze : Subsystem  TreatAsAtomicUnit=on
  wind speed : Outport
  wires:
  time freeze/1(out) -> Sum/2
  Constant/1 -> Switch/1
  Clock/1 -> time freeze/1(in), Compare To Constant/1, Sum/1, Switch/2
  Compare To Constant/1 -> 1-cos gust/Enable, time freeze/Trigger
  Sum/1 -> 1-cos gust/1(in)
  1-cos gust/1(wind) -> Switch/3
  Switch/1 -> wind speed/1

== system AircraftModel_LonMot_SAS/Test Sequences/SAS Test Sequence/Gust Generator ==
  1-cos gust : Subsystem  TreatAsAtomicUnit=on
  Clock : Clock
  Compare To Constant : simulink/Logic and Bit Operations/Compare To Constant  relop=>=  const=gust_start  OutDataTypeStr=boolean
  Constant : Constant  Value=0
  Sum : Sum  Inputs=+-|
  Switch : Switch  Criteria=u2 > Threshold  Threshold=gust_start+gust_duration  SaturateOnIntegerOverflow=off  InputSameDT=off
  time freeze : Subsystem  TreatAsAtomicUnit=on
  wind speed : Outport
  wires:
  time freeze/1(out) -> Sum/2
  Constant/1 -> Switch/1
  Clock/1 -> time freeze/1(in), Compare To Constant/1, Sum/1, Switch/2
  Compare To Constant/1 -> 1-cos gust/Enable, time freeze/Trigger
  Sum/1 -> 1-cos gust/1(in)
  1-cos gust/1(wind) -> Switch/3
  Switch/1 -> wind speed/1

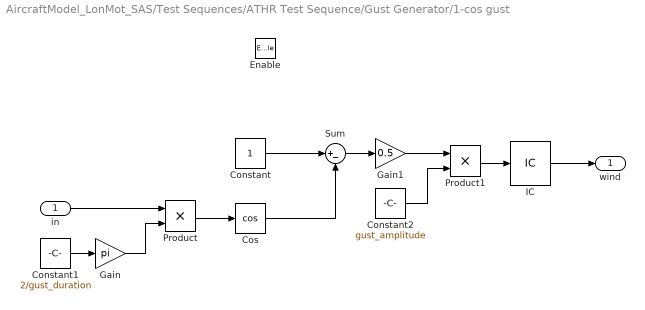
== system AircraftModel_LonMot_SAS/Test Sequences/ATHR Test Sequence/Gust Generator/1-cos gust ==
  in : Inport
  Enable : EnablePort  StatesWhenEnabling=reset
  Constant : Constant
  Constant1 : Constant  Value=2/gust_duration
  Constant2 : Constant  Value=gust_amplitude
  Cos : Trigonometry  Operator=cos
  Gain : Gain  Gain=pi
  Gain1 : Gain  Gain=0.5
  IC : InitialCondition  Value=0
  Product : Product
  Product1 : Product
  Sum : Sum  Inputs=|+-
  wind : Outport
  wires:
  IC/1 -> wind/1
  Constant1/1 -> Gain/1
  Product1/1 -> IC/1
  Product/1 -> Cos/1
  Cos/1 -> Sum/2
  Constant/1 -> Sum/1
  Gain/1 -> Product/2
  Gain1/1 -> Product1/1
  Sum/1 -> Gain1/1
  Constant2/1 -> Product1/2
  in/1 -> Product/1

== system AircraftModel_LonMot_SAS/Test Sequences/ATHR Test Sequence/Gust Generator/time freeze ==
  in : Inport
  Trigger : TriggerPort  VariantControl=Variant
  out : Outport  InitialOutput=0
  wires:
  in/1 -> out/1

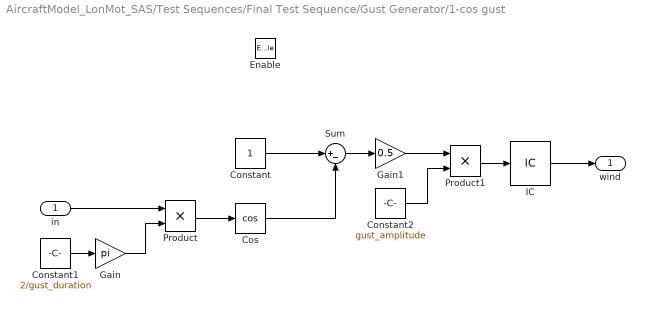
== system AircraftModel_LonMot_SAS/Test Sequences/Final Test Sequence/Gust Generator/1-cos gust ==
  in : Inport
  Enable : EnablePort  StatesWhenEnabling=reset
  Constant : Constant
  Constant1 : Constant  Value=2/gust_duration
  Constant2 : Constant  Value=gust_amplitude
  Cos : Trigonometry  Operator=cos
  Gain : Gain  Gain=pi
  Gain1 : Gain  Gain=0.5
  IC : InitialCondition  Value=0
  Product : Product
  Product1 : Product
  Sum : Sum  Inputs=|+-
  wind : Outport
  wires:
  IC/1 -> wind/1
  Constant1/1 -> Gain/1
  Product1/1 -> IC/1
  Product/1 -> Cos/1
  Cos/1 -> Sum/2
  Constant/1 -> Sum/1
  Gain/1 -> Product/2
  Gain1/1 -> Product1/1
  Sum/1 -> Gain1/1
  Constant2/1 -> Product1/2
  in/1 -> Product/1

== system AircraftModel_LonMot_SAS/Test Sequences/Final Test Sequence/Gust Generator/time freeze ==
  in : Inport
  Trigger : TriggerPort  VariantControl=Variant
  out : Outport  InitialOutput=0
  wires:
  in/1 -> out/1

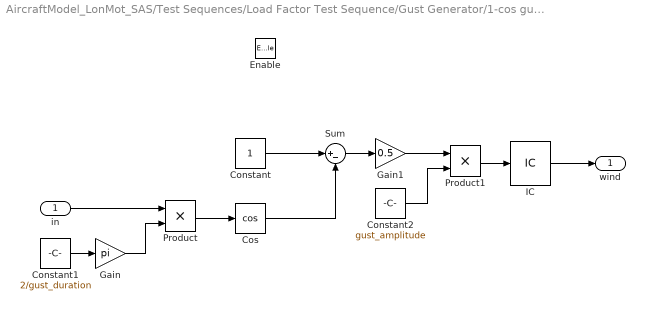
== system AircraftModel_LonMot_SAS/Test Sequences/Load Factor Test Sequence/Gust Generator/1-cos gust ==
  in : Inport
  Enable : EnablePort  StatesWhenEnabling=reset
  Constant : Constant
  Constant1 : Constant  Value=2/gust_duration
  Constant2 : Constant  Value=gust_amplitude
  Cos : Trigonometry  Operator=cos
  Gain : Gain  Gain=pi
  Gain1 : Gain  Gain=0.5
  IC : InitialCondition  Value=0
  Product : Product
  Product1 : Product
  Sum : Sum  Inputs=|+-
  wind : Outport
  wires:
  IC/1 -> wind/1
  Constant1/1 -> Gain/1
  Product1/1 -> IC/1
  Product/1 -> Cos/1
  Cos/1 -> Sum/2
  Constant/1 -> Sum/1
  Gain/1 -> Product/2
  Gain1/1 -> Product1/1
  Sum/1 -> Gain1/1
  Constant2/1 -> Product1/2
  in/1 -> Product/1

== system AircraftModel_LonMot_SAS/Test Sequences/Load Factor Test Sequence/Gust Generator/time freeze ==
  in : Inport
  Trigger : TriggerPort  VariantControl=Variant
  out : Outport  InitialOutput=0
  wires:
  in/1 -> out/1

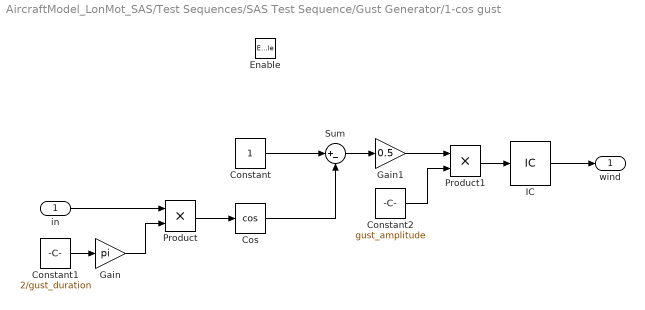
== system AircraftModel_LonMot_SAS/Test Sequences/SAS Test Sequence/Gust Generator/1-cos gust ==
  in : Inport
  Enable : EnablePort  StatesWhenEnabling=reset
  Constant : Constant
  Constant1 : Constant  Value=2/gust_duration
  Constant2 : Constant  Value=gust_amplitude
  Cos : Trigonometry  Operator=cos
  Gain : Gain  Gain=pi
  Gain1 : Gain  Gain=0.5
  IC : InitialCondition  Value=0
  Product : Product
  Product1 : Product
  Sum : Sum  Inputs=|+-
  wind : Outport
  wires:
  IC/1 -> wind/1
  Constant1/1 -> Gain/1
  Product1/1 -> IC/1
  Product/1 -> Cos/1
  Cos/1 -> Sum/2
  Constant/1 -> Sum/1
  Gain/1 -> Product/2
  Gain1/1 -> Product1/1
  Sum/1 -> Gain1/1
  Constant2/1 -> Product1/2
  in/1 -> Product/1

== system AircraftModel_LonMot_SAS/Test Sequences/SAS Test Sequence/Gust Generator/time freeze ==
  in : Inport
  Trigger : TriggerPort  VariantControl=Variant
  out : Outport  InitialOutput=0
  wires:
  in/1 -> out/1
